simulink model "Model_SinglePhase_TwoArm"  (R2022a)
settings: Solver=VariableStepAuto  StartTime=0.0  StopTime=10.0  RelTol=1e-3
libraries: fl_lib x13
settings Model: Creator=chack  LastModifiedBy=chack

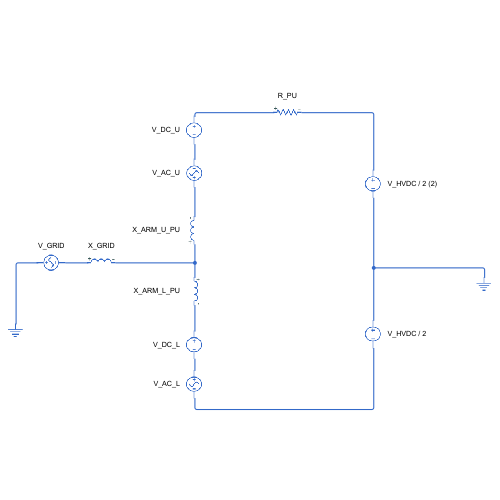
[thumbnail: Simulink's stored preview of the top-level diagram]
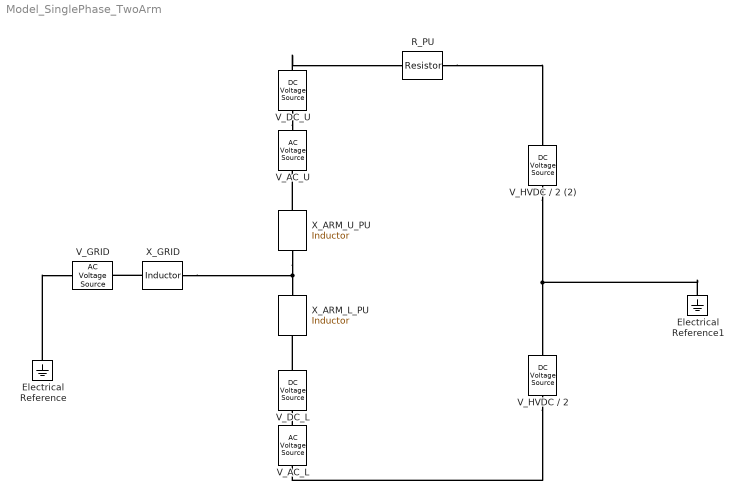
== system Model_SinglePhase_TwoArm ==
  Electrical Reference : fl_lib/Electrical/Electrical Elements/Electrical Reference
      settings: SourceProductBaseCode=PW,SS,VE
  Electrical Reference1 : fl_lib/Electrical/Electrical Elements/Electrical Reference
      settings: SourceProductBaseCode=PW,SS,VE
  R_PU : fl_lib/Electrical/Electrical Elements/Resistor  R=1 Ohm  i_specify=off  i_priority=None  i=0 A  i_nominal_specify=off  i_nominal_unit=A  i_nominal_value=1  v_specify=off  v_priority=None  v=0 V  v_nominal_specify=off  v_nominal_unit=V  v_nominal_value=1
      settings: SourceProductBaseCode=PW,SS,VE
  V_AC_L : fl_lib/Electrical/Electrical Sources/AC Voltage Source  amp=1 V  shift=0 deg  frequency=60 Hz  omega=0 rad/s
      settings: SourceProductBaseCode=PW,SS,VE
  V_AC_U : fl_lib/Electrical/Electrical Sources/AC Voltage Source  amp=1 V  shift=0 deg  frequency=60 Hz  omega=0 rad/s
      settings: SourceProductBaseCode=PW,SS,VE
  V_DC_L : fl_lib/Electrical/Electrical Sources/DC Voltage Source  v0=1 V
      settings: SourceProductBaseCode=PW,SS,VE
  V_DC_U : fl_lib/Electrical/Electrical Sources/DC Voltage Source  v0=1 V
      settings: SourceProductBaseCode=PW,SS,VE
  V_GRID : fl_lib/Electrical/Electrical Sources/AC Voltage Source  amp=1 V  shift=0 deg  frequency=60 Hz  omega=0 rad/s
      settings: SourceProductBaseCode=PW,SS,VE
  V_HVDC / 2 : fl_lib/Electrical/Electrical Sources/DC Voltage Source  v0=1 V
      settings: SourceProductBaseCode=PW,SS,VE
  V_HVDC / 2 (2) : fl_lib/Electrical/Electrical Sources/DC Voltage Source  v0=1 V
      settings: SourceProductBaseCode=PW,SS,VE
  X_ARM_L_PU : fl_lib/Electrical/Electrical Elements/Inductor  l=1e-6 H  r=0 Ohm  g=1e-9 1/Ohm  i_specify=off  i_priority=None  i=0 A  i_nominal_specify=off  i_nominal_unit=A  i_nominal_value=1  v_specify=off  v_priority=None  v=0 V  v_nominal_specify=off  v_nominal_unit=V  v_nominal_value=1  i_L_specify=off  i_L_priority=High  i_L=0 A  i_L_nominal_specify=off  i_L_nominal_unit=A  i_L_nominal_value=1
      settings: SourceProductBaseCode=PW,SS,VE
  X_ARM_U_PU : fl_lib/Electrical/Electrical Elements/Inductor  l=1e-6 H  r=0 Ohm  g=1e-9 1/Ohm  i_specify=off  i_priority=None  i=0 A  i_nominal_specify=off  i_nominal_unit=A  i_nominal_value=1  v_specify=off  v_priority=None  v=0 V  v_nominal_specify=off  v_nominal_unit=V  v_nominal_value=1  i_L_specify=off  i_L_priority=High  i_L=0 A  i_L_nominal_specify=off  i_L_nominal_unit=A  i_L_nominal_value=1
      settings: SourceProductBaseCode=PW,SS,VE
  X_GRID : fl_lib/Electrical/Electrical Elements/Inductor  l=1e-6 H  r=0 Ohm  g=1e-9 1/Ohm  i_specify=off  i_priority=None  i=0 A  i_nominal_specify=off  i_nominal_unit=A  i_nominal_value=1  v_specify=off  v_priority=None  v=0 V  v_nominal_specify=off  v_nominal_unit=V  v_nominal_value=1  i_L_specify=off  i_L_priority=High  i_L=0 A  i_L_nominal_specify=off  i_L_nominal_unit=A  i_L_nominal_value=1
      settings: SourceProductBaseCode=PW,SS,VE
  connections:
  X_ARM_U_PU/RConn1 -- V_AC_U/LConn1
  V_DC_U/RConn1 -- V_AC_U/RConn1
  X_ARM_U_PU/LConn1 -- X_GRID/RConn1 -- X_ARM_L_PU/LConn1
  X_GRID/LConn1 -- V_GRID/RConn1
  Electrical Reference/LConn1 -- V_GRID/LConn1
  V_DC_L/LConn1 -- X_ARM_L_PU/RConn1
  V_HVDC / 2 (2)/RConn1 -- Electrical Reference1/LConn1 -- V_HVDC / 2/LConn1
  V_DC_U/LConn1 -- R_PU/LConn1
  R_PU/RConn1 -- V_HVDC / 2 (2)/LConn1
  V_AC_L/LConn1 -- V_DC_L/RConn1
  V_HVDC / 2/RConn1 -- V_AC_L/RConn1
